simulink model "Q7_W1"  (R2020b)
settings: Solver=VariableStepAuto  StartTime=0.0  StopTime=10.0  RelTol=1e-3
settings Model: Creator=hp  LastModifiedBy=hp

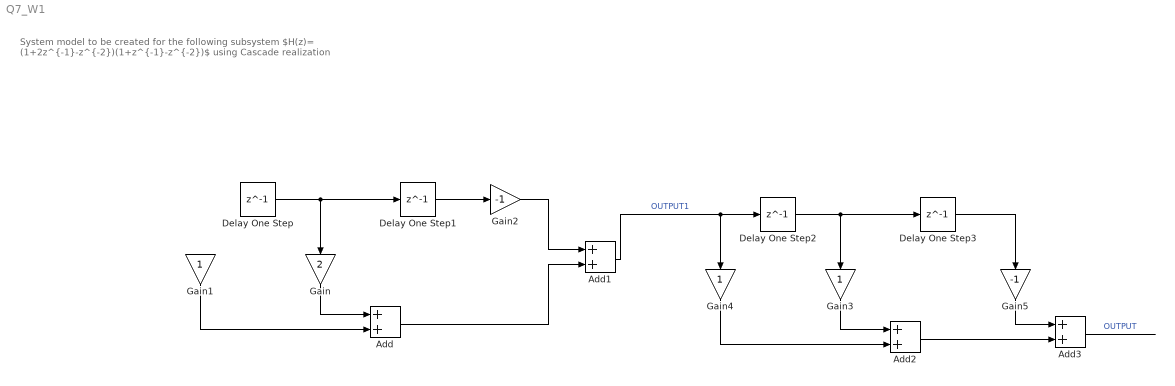
== system Q7_W1 ==
  note: System model to be created for the following subsystem
      | $H(z)= (1+2z^{-1}-z^{-2})(1+z^{-1}-z^{-2})$
      | using Cascade realization
  Add{,1..3} (4 alike) : Sum
  Delay One Step{,1..3} (4 alike) : Delay  DelayLength=1
  Gain : Gain  Gain=2
  Gain1 : Gain
  Gain2 : Gain  Gain=-1
  Gain3 : Gain
  Gain4 : Gain
  Gain5 : Gain  Gain=-1
  wires:
  ? -> Gain1/1, Delay One Step/1  "INPUT"
  Delay One Step/1 -> Delay One Step1/1, Gain/1
  Gain1/1 -> Add/2
  Gain/1 -> Add/1
  Delay One Step1/1 -> Gain2/1
  Add/1 -> Add1/2
  Gain2/1 -> Add1/1
  Add1/1 -> Gain4/1, Delay One Step2/1  "OUTPUT1"
  Delay One Step2/1 -> Delay One Step3/1, Gain3/1
  Delay One Step3/1 -> Gain5/1
  Gain3/1 -> Add2/1
  Gain4/1 -> Add2/2
  Add2/1 -> Add3/2
  Gain5/1 -> Add3/1
  Add3/1 -> ?  "OUTPUT"
